simulink model "simu_vent"  (R2018b)
settings: Solver=VariableStepAuto  StartTime=0.0  StopTime=4  RelTol=1e-3
values from neighbouring files (symbols this model uses):
  A = [-1699.79754719  0  0; 0  0  1; 4084.20094755  -134264.906868  -45.3800312243]    [params.mat]
  B = [584.53012025 0 0]    [params.mat]
  C = [0 1.00000000003 0]    [params.mat]
  D = 0    [params.mat]
  Klqi = lqi(sis,Q,R)    [ControladorMotor.m]    (also in params.mat = [1.84165907904 -53.1249874456 0.937627791744 -187.082869339]; ventilador.m)
settings Model: Creator=jacqu  LastModifiedBy=jacqu

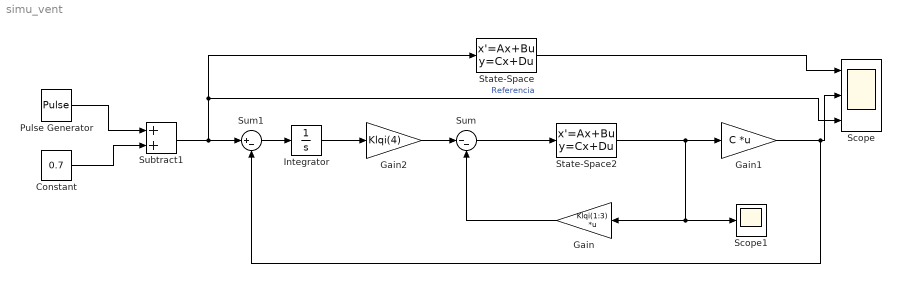
== system simu_vent ==
  Constant : Constant  Value=0.7
  Gain : Gain  Gain=Klqi(1:3)  Multiplication=Matrix(K*u) (u vector)
  Gain1 : Gain  Gain=C  Multiplication=Matrix(K*u) (u vector)
  Gain2 : Gain  Gain=Klqi(4)
  Integrator : Integrator
  Pulse Generator : DiscretePulseGenerator  PulseType=Time based  Amplitude=2  Period=1/0.5  PulseWidth=50
  Scope : Scope  NumInputPorts=3
  Scope1 : Scope
  State-Space : StateSpace  A=A  B=B  C=C  D=D  InitialCondition=0
  State-Space2 : StateSpace  A=A  B=B  C=eye(3)  D=zeros(3,1)  InitialCondition=0
  Subtract1 : Sum
  Sum : Sum  Inputs=|--
  Sum1 : Sum  Inputs=|+-
  wires:
  Constant/1 -> Subtract1/2
  Pulse Generator/1 -> Subtract1/1
  Subtract1/1 -> Scope/3, State-Space/1, Sum1/1  "Referencia"
  Gain/1 -> Sum/2
  State-Space/1 -> Scope/1
  Gain1/1 -> Sum1/2, Scope/2
  Sum/1 -> State-Space2/1
  State-Space2/1 -> Gain/1, Scope1/1, Gain1/1
  Sum1/1 -> Integrator/1
  Integrator/1 -> Gain2/1
  Gain2/1 -> Sum/1
